simulink model "twoStateMachineRiseFall"  (R2024b)
settings: Solver=VariableStepAuto  StartTime=0.0  StopTime=10.0  RelTol=1e-3
settings Model: Creator=optimus  LastModifiedBy=optimus
settings SFSimCC: SimTargetLang=C++

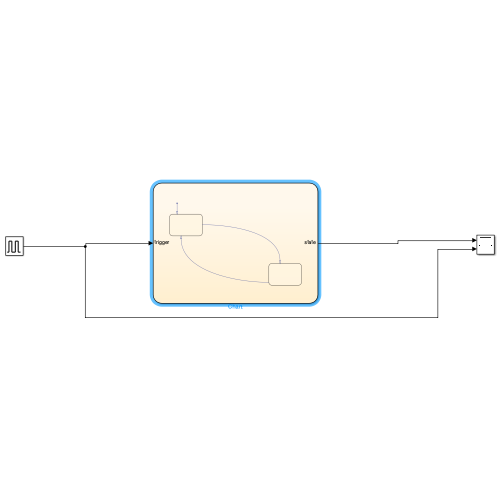
[thumbnail: Simulink's stored preview of the top-level diagram]
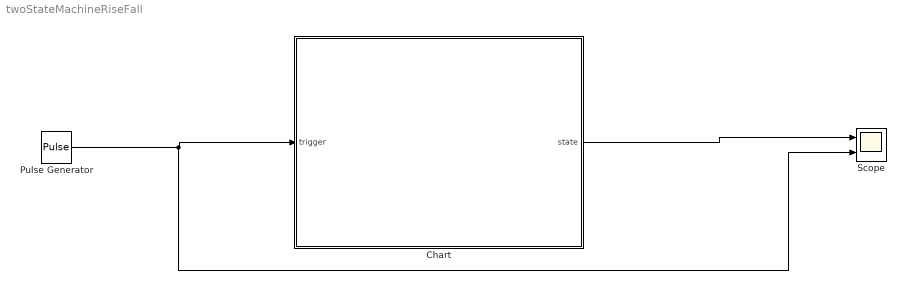
== system twoStateMachineRiseFall ==
  Chart : Stateflow chart  TreatAsAtomicUnit=on
  Pulse Generator : DiscretePulseGenerator  PulseType=Time based  PulseWidth=50
  Scope : Scope  NumInputPorts=2
  wires:
  Pulse Generator/1 -> Scope/2, Chart/1(trigger)
  Chart/1(state) -> Scope/1

== stateflow chart twoStateMachineRiseFall/Chart ==
  state Idle
    entry: state=0;
    prev=0;
  state Active
    entry: state=1;
    prev=1;
  (default) -> Idle
  Idle -> Active : [trigger==1 && prev==0]
  Active -> Idle : [trigger==0 && prev==1]
  data: trigger input; state output; prev local =0
